simulink model "JOEL"  (R2018a)
settings: Solver=FixedStepDiscrete  StartTime=0.0  StopTime=0.001  RelTol=1e-3
values from neighbouring files (symbols this model uses):
  fs = 20000    [filterbankProto.m]    (also in main.m = 44100)
undefined symbols (not defined in the file or in its folder): fdesignblkfcn, gcbh
libraries: dspsrcs4 x1, dspxfrm3 x1, dspobslib x1
settings Model: SimulationMode=accelerator  Creator=Kavi  LastModifiedBy=Kavi
settings SolverCC: AutoInsertRateTranBlk=on
settings DataIOCC: LimitDataPoints=on  SaveOutput=off  SignalLogging=off  SaveTime=off
settings OptimizationCC: LifeSpan=inf  SimCompilerOptimization=on
settings DebuggingCC: AlgebraicLoopMsg=error  SingleTaskRateTransMsg=error  AllowSymbolicDim=off  SFUnexpectedBacktrackingDiag=warning  SFNoUnconditionalDefaultTransitionDiag=warning  SFExecutionAtInitializationDiag=none
settings CodeAppCC: StateflowObjectComments=on
settings GRTTargetCC: TargetLangStandard=C89/C90 (ANSI)  GeneratePreprocessorConditionals=Disable all
settings ConfigComp: CovMetricSettings=dw  CovHtmlReporting=on  CovSaveCumulativeToWorkspaceVar=on  CovSaveSingleToWorkspaceVar=on  CovExternalEMLEnable=off  CovSFcnEnable=off

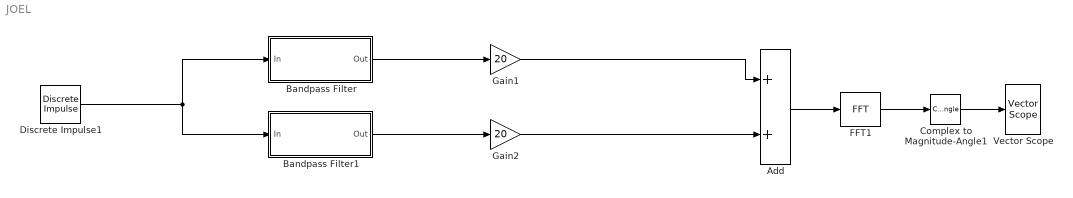
== system JOEL ==
  Add : Sum
  Bandpass Filter : Subsystem  DialogController=fdesignblkfcn  InitFcn=fdesignblkfcn(gcbh, {'InitFcn'});  mask(Bandpass Filter){}
      mask help: Design a bandpass filter
      settings: CopyFcn=fdesignblkfcn(gcbh, {'CopyFcn'});
      mask Help: helpview(mapfilelocation('dsp'), 'dspbandpassfilter');
      mask Display: disp('Bandpass');
  Bandpass Filter1 : Subsystem  DialogController=fdesignblkfcn  InitFcn=fdesignblkfcn(gcbh, {'InitFcn'});  mask(Bandpass Filter){}
      mask help: Design a bandpass filter
      settings: CopyFcn=fdesignblkfcn(gcbh, {'CopyFcn'});
      mask Help: helpview(mapfilelocation('dsp'), 'dspbandpassfilter');
      mask Display: disp('Bandpass');
  Complex to Magnitude-Angle1 : ComplexToMagnitudeAngle  Output=Magnitude
  Discrete Impulse1 : dspsrcs4/Discrete  Impulse  Delay=0  SampleTime=1/fs  FrameSample=512  OutputFrames=off  dataType=double  isSigned=on  wordLen=16  udDataType=sfix(16)  fracBitsMode=Best precision  numFracBits=15  OutDataTypeStr=double  LastOutDataTypeStr=double
  FFT1 : dspxfrm3/FFT  FFTImplementation=Auto  CompMethod=Table lookup  TableOpt=NEW  TableOptActive=Speed  BitRevOrder=off  Normalize=off  InheritFFTLength=on  FFTLength=64  WrapInput=on  roundingMode=Floor  overflowMode=off  firstCoeffDataTypeStr=Inherit: Same word length as input  firstCoeffLastDataTypeStr=Inherit: Same word length as input  outputMin=[]  outputMax=[]
  Gain1 : Gain  Gain=20
  Gain2 : Gain  Gain=20
  Vector Scope : dspobslib/Vector Scope  ScopeProperties=off  Domain=Frequency  HorizSpan=1  DisplayProperties=off  AxisGrid=on  Memory=off  FrameNumber=on  AxisLegend=off  AxisZoom=off  OpenScopeAtSimStart=on  OpenScopeImmediately=off  FigPos=[86 244 1118 420]  AxisProperties=on  XUnits=Hertz  XRange=[0...Fs/2]  InheritXIncr=on  XIncr=1  XLabel=Samples  XLimit=Auto  XMin=0  XMax=1  XStart=0  YUnits=dB  YLabel=|Magnitude (dB)|  LineProperties=off  LineStyles=-  LineMarkers=None  LineColors=[0 0 0]  XAxisParamsVer=6.9
      settings: SourceProductName=DSP System Toolbox  SourceProductBaseCode=DS  YMin=0.0723692553519949  YMax=69.3188381671759
  wires:
  Gain1/1 -> Add/1
  Bandpass Filter/1(Out) -> Gain1/1
  Discrete Impulse1/1 -> Bandpass Filter/1(In), Bandpass Filter1/1(In)
  Gain2/1 -> Add/2
  Add/1 -> FFT1/1
  Bandpass Filter1/1(Out) -> Gain2/1
  FFT1/1 -> Complex to Magnitude-Angle1/1
  Complex to Magnitude-Angle1/1 -> Vector Scope/1

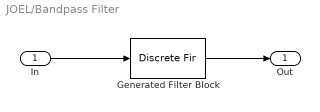
== system JOEL/Bandpass Filter ==
  In : Inport
  Generated Filter Block : DiscreteFir  Tag=BlockMethodSubSystem  Coefficients=[0.000639816347610437154 -0.000511300230993094349 -0.000312633337614588453 -0.000155768883099730309 -3.56834566911297751e-05 3.09827602980688695e-05 1.34581936856901235e-05 -0.000111082567480470944 -0.000334152920970287549 -0.000597596298732064085 -0.000796778369085952929 -0.000805062516806094499 -0.000519554617280051597 8.73325396986945993e-05 0.000927771727554775952 0.00179396059805746687 0.00239303116733106253 0.0024292172806776491 0.00170628117446267047 0.000225557930702637011 -0.00176053708552054806 -0.00376688099383176668 -0.00517677198195036752 -0.00540986738738212687 -0.00411651547974889453 -0.00133761119584771418 0.00242454337724467509 0.006269440390657844 0.00909508730372082796 0.00989440374699566971 0.00807397043790806374 0.00370065029215183115 -0.00240991497560243736 -0.00881475288598354556 -0.0137694846911104469 -0.0156889807306969872 -0.0136240722106269127 -0.00761847436612120028 0.00118156308040890442 0.0107105787239475444 0.0184694416009815732 0.0221641633224241019 0.0203764978016888337 0.0130452479088225617 0.00160485880564338731 -0.0112634104325683351 -0.0222628249538932288 -0.0283307697087098499 -0.0274942737703413806 -0.019480834505224396 -0.00591210945814074022 0.0100111981101771788 0.0242707550100718962 0.0330658488784100688 0.0338360692860983914 0.0260096602556506053 0.0112428824990210268 -0.00692656014462757121 -0.0239444087972972598 -0.0354081445886335125 -0.038230945894057955 -0.0314876938256120759 -0.0167081347032756143 0.00247726525227430668 0.0212505600278808972 0.0348492490234847616 0.0398044177237893287 0.0348492490234847616 0.0212505600278808972 0.00247726525227430668 -0.0167081347032756143 -0.0314876938256120759 -0.038230945894057955 -0.0354081445886335125 -0.0239444087972972598 -0.00692656014462757121 0.0112428824990210268 0.0260096602556506053 0.0338360692860983914 0.0330658488784100688 0.0242707550100718962 0.0100111981101771788 -0.00591210945814074022 -0.019480834505224396 -0.0274942737703413806 -0.0283307697087098499 -0.0222628249538932288 -0.0112634104325683351 0.00160485880564338731 0.0130452479088225617 0.0203764978016888337 0.0221641633224241019 0.0184694416009815732 0.0107105787239475444 0.00118156308040890442 -0.00761847436612120028 -0.0136240722106269127 -0.0156889807306969872 -0.0137694846911104469 -0.00881475288598354556 -0.00240991497560243736 0.00370065029215183115 0.00807397043790806374 0.00989440374699566971 0.00909508730372082796 0.006269440390657844 0.00242454337724467509 -0.00133761119584771418 -0.00411651547974889453 -0.00540986738738212687 -0.00517677198195036752 -0.00376688099383176668 -0.00176053708552054806 0.000225557930702637011 0.00170628117446267047 0.0024292172806776491 0.00239303116733106253 0.00179396059805746687 0.000927771727554775952 8.73325396986945993e-05 -0.000519554617280051597 -0.000805062516806094499 -0.000796778369085952929 -0.000597596298732064085 -0.000334152920970287549 -0.000111082567480470944 1.34581936856901235e-05 3.09827602980688695e-05 -3.56834566911297751e-05 -0.000155768883099730309 -0.000312633337614588453 -0.000511300230993094349 0.000639816347610437154]  InputProcessing=Columns as channels (frame based)
  Out : Outport
  wires:
  In/1 -> Generated Filter Block/1
  Generated Filter Block/1 -> Out/1

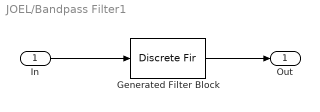
== system JOEL/Bandpass Filter1 ==
  In : Inport
  Generated Filter Block : DiscreteFir  Tag=BlockMethodSubSystem  Coefficients=[0.000638808451681908821 -2.83262166050421297e-05 -0.000873949528954946417 -0.00158946310796689578 -0.00121892459966629375 0.000534699838326503944 0.00266146987282030525 0.00330259721976598189 0.00128091953120987052 -0.00251090104086588647 -0.00529900129071889277 -0.00446366036512952161 5.69476295421665613e-05 0.00520415019324160181 0.00695536159683846859 0.00367340222859283095 -0.00227586316996280982 -0.0063155523005638415 -0.00553867771932096183 -0.00121439240354370031 0.00252981785562487928 0.00277933580878940824 0.000720068979309173608 0.000232197608414970653 0.00324012706675185077 0.00656153168133619385 0.0042495906033136379 -0.00579516914342536466 -0.0172328840380182487 -0.0185472273112479609 -0.0032449960988308298 0.0214502994484101553 0.0366976507879190478 0.0260094790013173129 -0.00902189276025771106 -0.0454114433135040518 -0.0537023413864879673 -0.0216311202866367146 0.0324552855022009895 0.0696422794283241831 0.0589799791661624745 0.0032047982476325447 -0.0598084417842409746 -0.0834548510487914397 -0.0477897023070045432 0.0236366112530307926 0.0797832260581755326 0.0797832260581755326 0.0236366112530307926 -0.0477897023070045432 -0.0834548510487914397 -0.0598084417842409746 0.0032047982476325447 0.0589799791661624745 0.0696422794283241831 0.0324552855022009895 -0.0216311202866367146 -0.0537023413864879673 -0.0454114433135040518 -0.00902189276025771106 0.0260094790013173129 0.0366976507879190478 0.0214502994484101553 -0.0032449960988308298 -0.0185472273112479609 -0.0172328840380182487 -0.00579516914342536466 0.0042495906033136379 0.00656153168133619385 0.00324012706675185077 0.000232197608414970653 0.000720068979309173608 0.00277933580878940824 0.00252981785562487928 -0.00121439240354370031 -0.00553867771932096183 -0.0063155523005638415 -0.00227586316996280982 0.00367340222859283095 0.00695536159683846859 0.00520415019324160181 5.69476295421665613e-05 -0.00446366036512952161 -0.00529900129071889277 -0.00251090104086588647 0.00128091953120987052 0.00330259721976598189 0.00266146987282030525 0.000534699838326503944 -0.00121892459966629375 -0.00158946310796689578 -0.000873949528954946417 -2.83262166050421297e-05 0.000638808451681908821]  InputProcessing=Columns as channels (frame based)
  Out : Outport
  wires:
  In/1 -> Generated Filter Block/1
  Generated Filter Block/1 -> Out/1
